simulink model "test_vannne_diverter"  (R2016a)
settings: Solver=FixedStepAuto  StartTime=0.0  StopTime=1000.0  RelTol=1e-3
undefined symbols (not defined in the file or in its folder): DiscIntNeverNeededParam
settings Model: Creator=frederic.amblard  LastModifiedBy=frederic.amblard

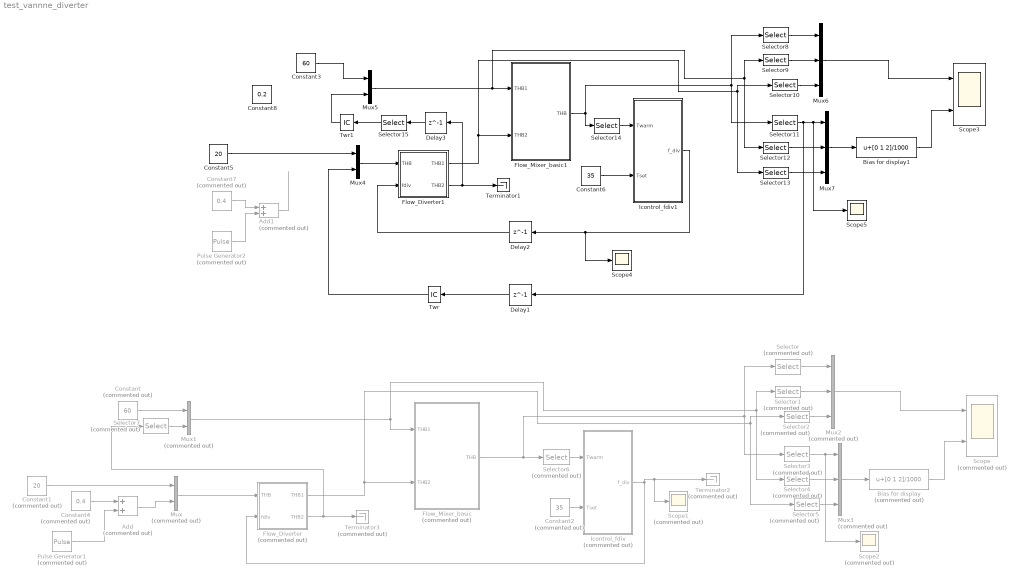
== system test_vannne_diverter ==
  Add : Sum  Commented=on
  Add1 : Sum  Commented=on
  Bias for display : Bias  Commented=on  Bias=[0 1 2]/1000
  Bias for display1 : Bias  Bias=[0 1 2]/1000
  Constant : Constant  Commented=on  Value=60
  Constant1 : Constant  Commented=on  Value=20
  Constant2 : Constant  Commented=on  Value=35
  Constant3 : Constant  Value=60
  Constant4 : Constant  Commented=on  Value=0.4
  Constant5 : Constant  Value=20
  Constant6 : Constant  Value=35
  Constant7 : Constant  Commented=on  Value=0.4
  Constant8 : Constant  Value=0.2
  Delay1 : Delay  DelayLength=1
  Delay2 : Delay  DelayLength=1
  Delay3 : Delay  DelayLength=1
  Flow_Diverter : Subsystem  Commented=on  AncestorBlock=carnot/Hydraulics/Flow_Diverter  mask(flow diverter, fixed rate){}
      mask help:
      | The block diverts an incoming massflow according to:
      | mdot1 = mdot * fdiv
      | mdot2 = mdot * (1-fdiv)
      | fdiv is limited to the range [0..1]
      mask Help: web(fullfile(path_carnot('help'),'Flow_Diverter.html'),'-helpbrowser')
      mask Display: plot(0,-5,120,65,[20 45 20 20],[20 30 40 20],[45 70 70 45],[30 20 40 30],[45 35 55 45],[30 10 10 30])
  Flow_Diverter1 : Subsystem  AncestorBlock=carnot/Hydraulics/Flow_Diverter  mask(flow diverter, fixed rate){}
      mask help:
      | The block diverts an incoming massflow according to:
      | mdot1 = mdot * fdiv
      | mdot2 = mdot * (1-fdiv)
      | fdiv is limited to the range [0..1]
      mask Help: web(fullfile(path_carnot('help'),'Flow_Diverter.html'),'-helpbrowser')
      mask Display: plot(0,-5,120,65,[20 45 20 20],[20 30 40 20],[45 70 70 45],[30 20 40 30],[45 35 55 45],[30 10 10 30])
  Flow_Mixer_basic : Subsystem  Commented=on  mask(Flow Mixer Basic){}
      mask help:
      | The flow mixer calculated the temperature and massflow of 2 entering flows.
      | The temperature is calculated in the block Mix_T_Mdot.
      | The flow diversion fdiv (feed back to the flow diverter) takes care that the pressure drop in the 2 branches is the same. The resulting pressure drop coefficients are calulated in the s-function mix_flow (uses solve_quadratic_equation in Carlib).
      mask Help: web(fullfile(path_carnot('help'),'Flow_Mixer_basic.html'),'-helpbrowser')
      mask Display: disp('Flow\nMixer')
  Flow_Mixer_basic1 : Subsystem  mask(Flow Mixer Basic){}
      mask help:
      | The flow mixer calculated the temperature and massflow of 2 entering flows.
      | The temperature is calculated in the block Mix_T_Mdot.
      | The flow diversion fdiv (feed back to the flow diverter) takes care that the pressure drop in the 2 branches is the same. The resulting pressure drop coefficients are calulated in the s-function mix_flow (uses solve_quadratic_equation in Carlib).
      mask Help: web(fullfile(path_carnot('help'),'Flow_Mixer_basic.html'),'-helpbrowser')
      mask Display: disp('Flow\nMixer')
  Icontrol_fdiv : Subsystem  Commented=on  AncestorBlock=carnot/Hydraulics/Flow_Mixer_Thermostatic/Icontrol_fdiv
  Icontrol_fdiv1 : Subsystem  AncestorBlock=carnot/Hydraulics/Flow_Mixer_Thermostatic/Icontrol_fdiv
  Mux : Mux  Commented=on  Inputs=2
  Mux1 : Mux  Commented=on  Inputs=2
  Mux2 : Mux  Commented=on  Inputs=3
  Mux3 : Mux  Commented=on  Inputs=3
  Mux4 : Mux  Inputs=2
  Mux5 : Mux  Inputs=2
  Mux6 : Mux  Inputs=3
  Mux7 : Mux  Inputs=3
  Pulse Generator1 : DiscretePulseGenerator  Commented=on  Amplitude=0.1  Period=100  PulseWidth=50
  Pulse Generator2 : DiscretePulseGenerator  Commented=on  Amplitude=0.1  Period=100  PulseWidth=50
  Scope : Scope  Commented=on  NumInputPorts=2
  Scope1 : Scope  Commented=on
  Scope2 : Scope  Commented=on
  Scope3 : Scope  NumInputPorts=2
  Scope4 : Scope
  Scope5 : Scope
  Selector{,1..2,6} (4 alike) : Selector  Commented=on  InputPortWidth=2  IndexOptions=Index vector (dialog)  Indices=[1]  OutputSizes=1
  Selector{8..10,14} (4 alike) : Selector  InputPortWidth=2  IndexOptions=Index vector (dialog)  Indices=[1]  OutputSizes=1
  Selector{11..13,15} (4 alike) : Selector  InputPortWidth=2  IndexOptions=Index vector (dialog)  Indices=[2]  OutputSizes=1
  Selector{3..5,7} (4 alike) : Selector  Commented=on  InputPortWidth=2  IndexOptions=Index vector (dialog)  Indices=[2]  OutputSizes=1
  Terminator1 : Terminator
  Terminator2 : Terminator  Commented=on
  Terminator3 : Terminator  Commented=on
  Twr : InitialCondition  Value=0.5
  Twr1 : InitialCondition  Value=0.2
  wires:
  Mux1/1 -> Flow_Mixer_basic/1(THB1), Selector4/1, Selector1/1
  Flow_Diverter/1(THB1) -> Selector5/1, Selector2/1, Flow_Mixer_basic/2(THB2)
  Flow_Mixer_basic/1(THB) -> Selector6/1, Selector3/1, Selector/1
  Mux2/1 -> Scope/1
  Mux3/1 -> Bias for display/1
  Bias for display/1 -> Scope/2
  Selector6/1 -> Icontrol_fdiv/1(Twarm)
  Constant2/1 -> Icontrol_fdiv/2(Tset)
  Constant1/1 -> Mux/1
  Mux/1 -> Flow_Diverter/1(THB)
  Flow_Diverter/2(THB2) -> Selector7/1, Terminator3/1
  Icontrol_fdiv/1(f_div) -> Scope1/1, Terminator2/1, Flow_Diverter/2(fdiv)
  Constant4/1 -> Add/1
  Constant/1 -> Mux1/1
  Selector7/1 -> Mux1/2
  Selector/1 -> Mux2/1
  Selector1/1 -> Mux2/2
  Selector2/1 -> Mux2/3
  Selector3/1 -> Scope2/1, Mux3/1
  Selector4/1 -> Mux3/2
  Selector5/1 -> Mux3/3
  Add/1 -> Mux/2
  Pulse Generator1/1 -> Add/2
  Mux5/1 -> Flow_Mixer_basic1/1(THB1), Selector12/1, Selector9/1
  Flow_Diverter1/1(THB1) -> Selector13/1, Selector10/1, Flow_Mixer_basic1/2(THB2)
  Flow_Mixer_basic1/1(THB) -> Selector14/1, Selector11/1, Selector8/1
  Mux6/1 -> Scope3/1
  Mux7/1 -> Bias for display1/1
  Bias for display1/1 -> Scope3/2
  Selector14/1 -> Icontrol_fdiv1/1(Twarm)
  Constant6/1 -> Icontrol_fdiv1/2(Tset)
  Constant5/1 -> Mux4/1
  Mux4/1 -> Flow_Diverter1/1(THB)
  Constant7/1 -> Add1/1
  Constant3/1 -> Mux5/1
  Selector9/1 -> Mux6/2
  Selector10/1 -> Mux6/3
  Selector12/1 -> Mux7/2
  Selector13/1 -> Mux7/3
  Add1/1 -> ?
  Pulse Generator2/1 -> Add1/2
  Selector11/1 -> Delay1/1, Scope5/1, Mux7/1
  Flow_Diverter1/2(THB2) -> Delay3/1, Terminator1/1
  Selector8/1 -> Mux6/1
  Icontrol_fdiv1/1(f_div) -> Delay2/1, Scope4/1
  Delay1/1 -> Twr/1
  Delay2/1 -> Flow_Diverter1/2(fdiv)
  Twr/1 -> Mux4/2
  Twr1/1 -> Mux5/2
  Selector15/1 -> Twr1/1
  Delay3/1 -> Selector15/1

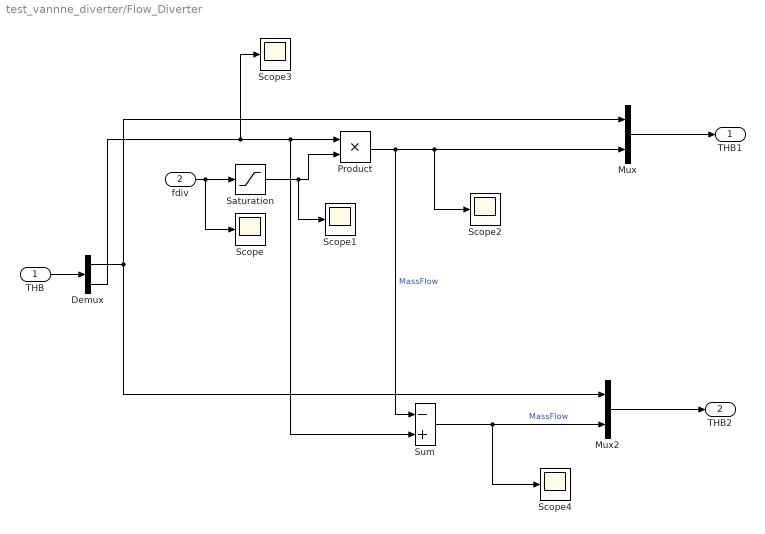
== system test_vannne_diverter/Flow_Diverter ==
  THB : Inport
  fdiv : Inport  Port=2
  Demux : Demux  Outputs=2
  Mux : Mux  Inputs=2
  Mux2 : Mux  Inputs=2
  Product : Product
  Saturation : Saturate  UpperLimit=1  LowerLimit=0
  Scope{,1..4} (5 alike) : Scope
  Sum : Sum  Inputs=-+  SaturateOnIntegerOverflow=on  InputSameDT=on  OutDataTypeStr=Inherit: Same as first input
  THB1 : Outport
  THB2 : Outport  Port=2
  wires:
  Saturation/1 -> Product/2, Scope1/1
  Sum/1 -> Scope4/1, Mux2/2  "MassFlow"
  Demux/2 -> Scope3/1, Product/1, Sum/2
  fdiv/1 -> Scope/1, Saturation/1
  Product/1 -> Sum/1, Scope2/1, Mux/2  "MassFlow"
  Mux/1 -> THB1/1
  Mux2/1 -> THB2/1
  THB/1 -> Demux/1
  Demux/1 -> Mux/1, Mux2/1

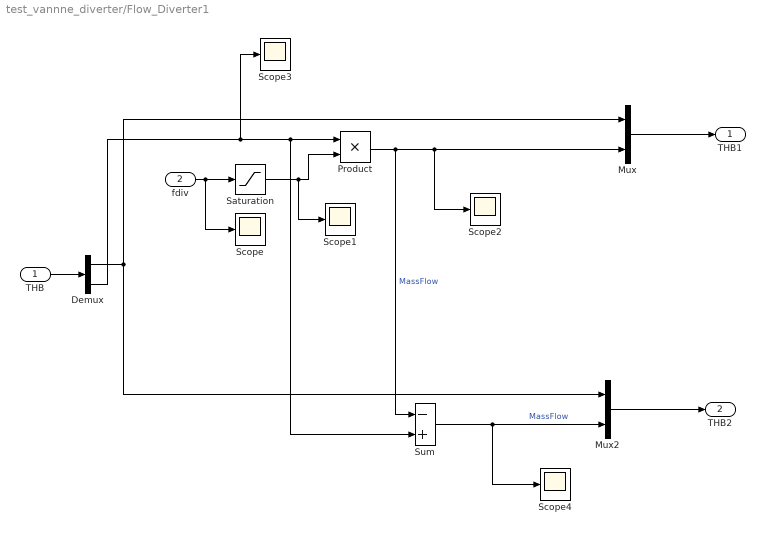
== system test_vannne_diverter/Flow_Diverter1 ==
  THB : Inport
  fdiv : Inport  Port=2
  Demux : Demux  Outputs=2
  Mux : Mux  Inputs=2
  Mux2 : Mux  Inputs=2
  Product : Product
  Saturation : Saturate  UpperLimit=1  LowerLimit=0
  Scope{,1..4} (5 alike) : Scope
  Sum : Sum  Inputs=-+  SaturateOnIntegerOverflow=on  InputSameDT=on  OutDataTypeStr=Inherit: Same as first input
  THB1 : Outport
  THB2 : Outport  Port=2
  wires:
  Saturation/1 -> Product/2, Scope1/1
  Sum/1 -> Scope4/1, Mux2/2  "MassFlow"
  Demux/2 -> Scope3/1, Product/1, Sum/2
  fdiv/1 -> Scope/1, Saturation/1
  Product/1 -> Sum/1, Scope2/1, Mux/2  "MassFlow"
  Mux/1 -> THB1/1
  Mux2/1 -> THB2/1
  THB/1 -> Demux/1
  Demux/1 -> Mux/1, Mux2/1

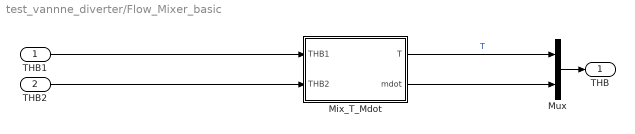
== system test_vannne_diverter/Flow_Mixer_basic ==
  THB1 : Inport
  THB2 : Inport  Port=2
  Mix_T_Mdot : Subsystem  mask(mix_temperature){mixcalc=Tmix = (mdot1*T1 + mdot2*T2)/(mdot1+mdot2)}
      mask prompts: mixcalc "Calculation of mixture :"
      mask help:
      | Calculate the temperature of the mixture of two flows. Uses enthalpy balance for humid air. Liquids may be mixed by the (faster and approximate) equation:
      | Tmix = (mdot1*T1 + mdot2*T2)/(mdot1+mdot2)
      mask Help: web(fullfile(path_carnot('help'),'Mix_T_Mdot.html'),'-helpbrowser')
      mask TypeOptions mixcalc: Tmix = (mdot1*T1 + mdot2*T2)/(mdot1+mdot2) | Enthalpy balance
  Mux : Mux  Inputs=2
  THB : Outport
  wires:
  THB1/1 -> Mix_T_Mdot/1(THB1)
  THB2/1 -> Mix_T_Mdot/2(THB2)
  Mix_T_Mdot/1(T) -> Mux/1  "T"
  Mix_T_Mdot/2(mdot) -> Mux/2
  Mux/1 -> THB/1

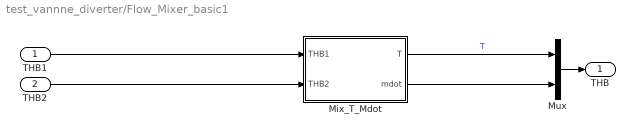
== system test_vannne_diverter/Flow_Mixer_basic1 ==
  THB1 : Inport
  THB2 : Inport  Port=2
  Mix_T_Mdot : Subsystem  mask(mix_temperature){mixcalc=Tmix = (mdot1*T1 + mdot2*T2)/(mdot1+mdot2)}
      mask prompts: mixcalc "Calculation of mixture :"
      mask help:
      | Calculate the temperature of the mixture of two flows. Uses enthalpy balance for humid air. Liquids may be mixed by the (faster and approximate) equation:
      | Tmix = (mdot1*T1 + mdot2*T2)/(mdot1+mdot2)
      mask Help: web(fullfile(path_carnot('help'),'Mix_T_Mdot.html'),'-helpbrowser')
      mask TypeOptions mixcalc: Tmix = (mdot1*T1 + mdot2*T2)/(mdot1+mdot2) | Enthalpy balance
  Mux : Mux  Inputs=2
  THB : Outport
  wires:
  THB1/1 -> Mix_T_Mdot/1(THB1)
  THB2/1 -> Mix_T_Mdot/2(THB2)
  Mix_T_Mdot/1(T) -> Mux/1  "T"
  Mix_T_Mdot/2(mdot) -> Mux/2
  Mux/1 -> THB/1

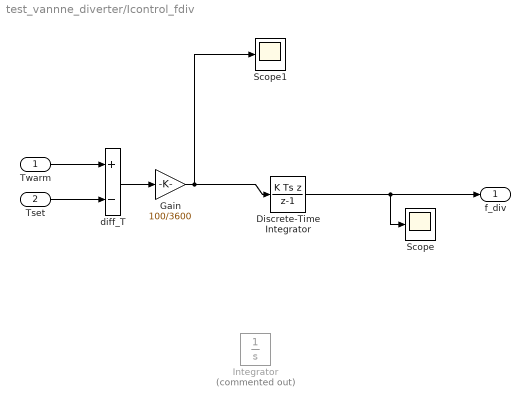
== system test_vannne_diverter/Icontrol_fdiv ==
  Twarm : Inport
  Tset : Inport  Port=2
  Discrete-Time Integrator : DiscreteIntegrator  IntegratorMethod=Integration: Backward Euler  InitialCondition=1  InitialConditionSetting=State (most efficient)  SampleTime=-1  LimitOutput=on  UpperSaturationLimit=1  LowerSaturationLimit=0  IgnoreLimit=on  ICPrevOutput=DiscIntNeverNeededParam  ICPrevScaledInput=DiscIntNeverNeededParam
  Gain : Gain  Gain=100/3600  SaturateOnIntegerOverflow=on  OutDataTypeStr=Inherit: Same as input  ParamDataTypeStr=Inherit: Same as input
  Integrator : Integrator  Commented=on  LimitOutput=on  UpperSaturationLimit=1  LowerSaturationLimit=0  ZeroCross=off
  Scope : Scope
  Scope1 : Scope
  diff_T : Sum  Inputs=+-  SaturateOnIntegerOverflow=on  InputSameDT=on  OutDataTypeStr=Inherit: Same as first input
  f_div : Outport
  wires:
  diff_T/1 -> Gain/1
  Twarm/1 -> diff_T/1
  Tset/1 -> diff_T/2
  Discrete-Time Integrator/1 -> f_div/1, Scope/1
  Gain/1 -> Scope1/1, Discrete-Time Integrator/1

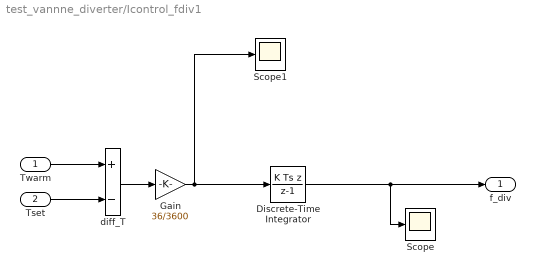
== system test_vannne_diverter/Icontrol_fdiv1 ==
  Twarm : Inport
  Tset : Inport  Port=2
  Discrete-Time Integrator : DiscreteIntegrator  IntegratorMethod=Integration: Backward Euler  InitialCondition=1  InitialConditionSetting=State (most efficient)  LimitOutput=on  UpperSaturationLimit=1  LowerSaturationLimit=0  IgnoreLimit=on  ICPrevOutput=DiscIntNeverNeededParam  ICPrevScaledInput=DiscIntNeverNeededParam
  Gain : Gain  Gain=36/3600  SaturateOnIntegerOverflow=on  OutDataTypeStr=Inherit: Same as input  ParamDataTypeStr=Inherit: Same as input
  Scope : Scope
  Scope1 : Scope
  diff_T : Sum  Inputs=+-  SaturateOnIntegerOverflow=on  InputSameDT=on  OutDataTypeStr=Inherit: Same as first input
  f_div : Outport
  wires:
  diff_T/1 -> Gain/1
  Twarm/1 -> diff_T/1
  Tset/1 -> diff_T/2
  Discrete-Time Integrator/1 -> Scope/1, f_div/1
  Gain/1 -> Scope1/1, Discrete-Time Integrator/1

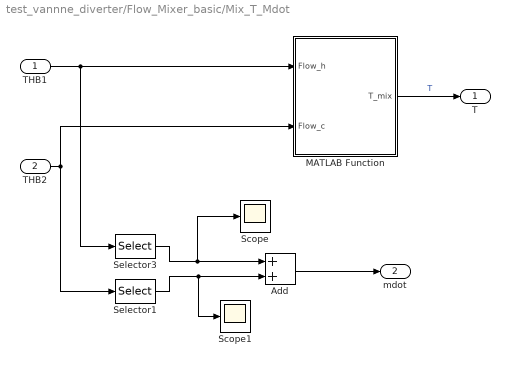
== system test_vannne_diverter/Flow_Mixer_basic/Mix_T_Mdot ==
  THB1 : Inport
  THB2 : Inport  Port=2
  Add : Sum
  MATLAB Function : MATLAB Function  TreatAsAtomicUnit=on
  Scope : Scope
  Scope1 : Scope
  Selector1 : Selector  InputPortWidth=2  IndexOptions=Index vector (dialog)  Indices=[2]  OutputSizes=1
  Selector3 : Selector  InputPortWidth=2  IndexOptions=Index vector (dialog)  Indices=[2]  OutputSizes=1
  T : Outport
  mdot : Outport  Port=2
  wires:
  Add/1 -> mdot/1
  Selector1/1 -> Scope1/1, Add/2
  MATLAB Function/1(T_mix) -> T/1  "T"
  THB1/1 -> MATLAB Function/1(Flow_h), Selector3/1
  THB2/1 -> MATLAB Function/2(Flow_c), Selector1/1
  Selector3/1 -> Scope/1, Add/1

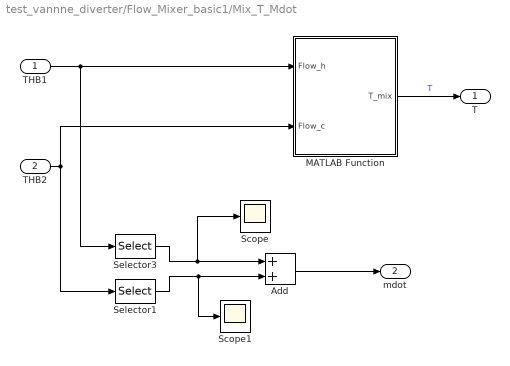
== system test_vannne_diverter/Flow_Mixer_basic1/Mix_T_Mdot ==
  THB1 : Inport
  THB2 : Inport  Port=2
  Add : Sum
  MATLAB Function : MATLAB Function  TreatAsAtomicUnit=on
  Scope : Scope
  Scope1 : Scope
  Selector1 : Selector  InputPortWidth=2  IndexOptions=Index vector (dialog)  Indices=[2]  OutputSizes=1
  Selector3 : Selector  InputPortWidth=2  IndexOptions=Index vector (dialog)  Indices=[2]  OutputSizes=1
  T : Outport
  mdot : Outport  Port=2
  wires:
  Add/1 -> mdot/1
  Selector1/1 -> Scope1/1, Add/2
  MATLAB Function/1(T_mix) -> T/1  "T"
  THB1/1 -> MATLAB Function/1(Flow_h), Selector3/1
  THB2/1 -> MATLAB Function/2(Flow_c), Selector1/1
  Selector3/1 -> Scope/1, Add/1

== matlab function test_vannne_diverter/Flow_Mixer_basic/Mix_T_Mdot/MATLAB Function ==
  data: Flow_h input; Flow_c input; T_mix output size=[1]
function T_mix  = mix_temperature(Flow_h , Flow_c)

T1 = Flow_h(1);
T2 = Flow_c(1);

MDOT1 = Flow_h(2);
MDOT2 = Flow_c(2);
mdotsum = MDOT1+MDOT2;
NO_MASSFLOW = 0;
    
if mdotsum < NO_MASSFLOW      % if sum of massflows < limit: no massflow
    T_mix = 0.5*(T1+T2);        % average temperature 
elseif MDOT2 < NO_MASSFLOW    % else if massflow in path 2 < limit
    T_mix = T1;
elseif MDOT1 < NO_MASSFLOW   % else if massflow in path 1 < limit */
    T_mix = T2;
else                          % both pathes open */
    T_mix = (MDOT1*T1+MDOT2*T2)/mdotsum;
end
end

== matlab function test_vannne_diverter/Flow_Mixer_basic1/Mix_T_Mdot/MATLAB Function ==
  data: Flow_h input; Flow_c input; T_mix output size=[1]
function T_mix  = mix_temperature(Flow_h , Flow_c)

T1 = Flow_h(1);
T2 = Flow_c(1);

MDOT1 = Flow_h(2);
MDOT2 = Flow_c(2);
mdotsum = MDOT1+MDOT2;
NO_MASSFLOW = 0;
    
if mdotsum < NO_MASSFLOW      % if sum of massflows < limit: no massflow
    T_mix = 0.5*(T1+T2);        % average temperature 
elseif MDOT2 < NO_MASSFLOW    % else if massflow in path 2 < limit
    T_mix = T1;
elseif MDOT1 < NO_MASSFLOW   % else if massflow in path 1 < limit */
    T_mix = T2;
else                          % both pathes open */
    T_mix = (MDOT1*T1+MDOT2*T2)/mdotsum;
end
end
